simulink model "hnn_with_proof"  (R2024b)
settings: Solver=VariableStepAuto  StartTime=0.0  StopTime=10.0  RelTol=1e-3
settings Model: Creator=merlin  LastModifiedBy=merlin

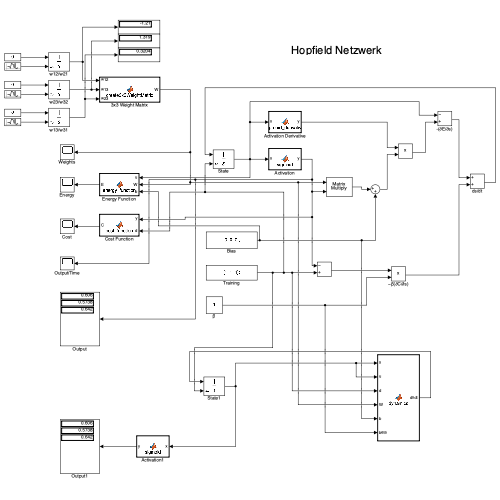
[thumbnail: Simulink's stored preview of the top-level diagram]
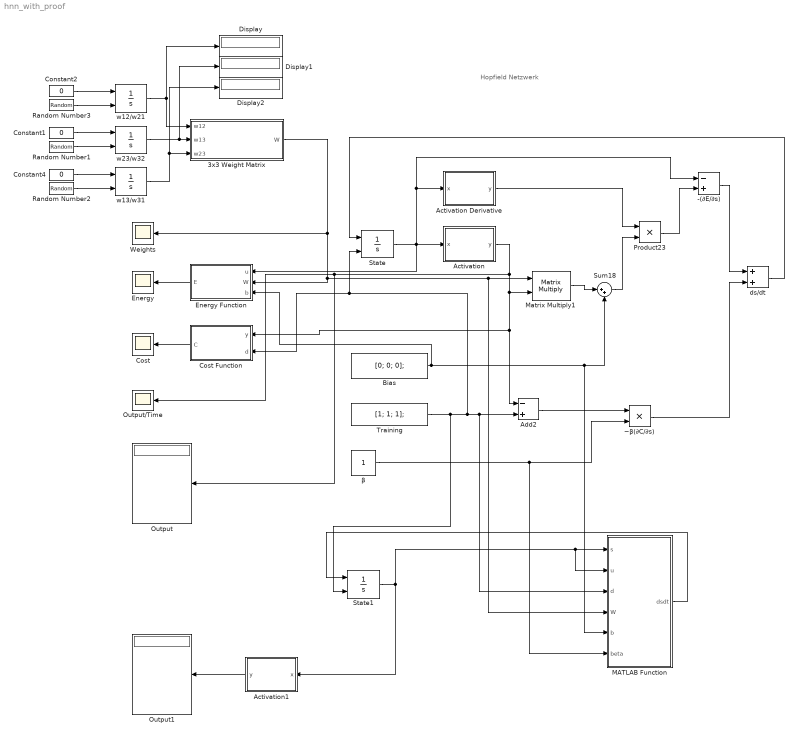
== system hnn_with_proof ==
  note: Hopfield Netzwerk
  -(∂E/∂s) : Sum  Inputs=-+
  3x3 Weight Matrix : MATLAB Function  TreatAsAtomicUnit=on
  Activation : MATLAB Function  TreatAsAtomicUnit=on
  Activation Derivative : MATLAB Function  TreatAsAtomicUnit=on
  Activation1 : MATLAB Function  TreatAsAtomicUnit=on
  Add2 : Sum  Inputs=-+
  Bias : Constant  Value=[0; 0; 0];  VectorParams1D=off
  Constant1 : Constant  Value=0
  Constant2 : Constant  Value=0
  Constant4 : Constant  Value=0
  Cost : Scope
  Cost Function : MATLAB Function  TreatAsAtomicUnit=on
  Display : Display
  Display1 : Display
  Display2 : Display
  Energy : Scope
  Energy Function : MATLAB Function  TreatAsAtomicUnit=on
  MATLAB Function : MATLAB Function  TreatAsAtomicUnit=on
  Matrix Multiply1 : Product  Multiplication=Matrix(*)
  Output : Display
  Output/Time : Scope
  Output1 : Display
  Product23 : Product
  Random Number1 : RandomNumber  Seed=23  SampleTime=0.1
  Random Number2 : RandomNumber  Seed=13  SampleTime=0.1
  Random Number3 : RandomNumber  Seed=12  SampleTime=0.1
  State : Integrator  InitialConditionSource=external
  State1 : Integrator  InitialConditionSource=external
  Sum18 : Sum  Inputs=|++
  Training : Constant  Value=[1; 1; 1];  VectorParams1D=off
  Weights : Scope
  ds/dt : Sum
  w12/w21 : Integrator  InitialConditionSource=external
  w13/w31 : Integrator  InitialConditionSource=external
  w23/w32 : Integrator  InitialConditionSource=external
  β : Constant  VectorParams1D=off
  −β(∂C/∂s) : Product
  wires:
  w12/w21/1 -> 3x3 Weight Matrix/1(w12), Display/1
  Constant4/1 -> w13/w31/1
  Random Number2/1 -> w13/w31/2
  Bias/1 -> MATLAB Function/5(b), Sum18/2, Energy Function/3(b)
  ds/dt/1 -> State/1
  Energy Function/1(E) -> Energy/1
  State/1 -> Activation/1(x), Energy Function/1(u), Activation Derivative/1(x), -(∂E/∂s)/1
  β/1 -> MATLAB Function/6(beta), −β(∂C/∂s)/2
  Training/1 -> State1/2, Cost Function/2(d), State/2, MATLAB Function/3(d), Add2/2
  Activation/1(y) -> Output/Time/1, Output/1, Cost Function/1(y), Add2/1, Matrix Multiply1/2
  -(∂E/∂s)/1 -> ds/dt/1
  Add2/1 -> −β(∂C/∂s)/1
  Matrix Multiply1/1 -> Sum18/1
  Activation Derivative/1(y) -> Product23/1
  Sum18/1 -> Product23/2
  −β(∂C/∂s)/1 -> ds/dt/2
  Cost Function/1(C) -> Cost/1
  Product23/1 -> -(∂E/∂s)/2
  3x3 Weight Matrix/1(W) -> Weights/1, Energy Function/2(W), MATLAB Function/4(W), Matrix Multiply1/1
  Constant2/1 -> w12/w21/1
  Random Number3/1 -> w12/w21/2
  Constant1/1 -> w23/w32/1
  Random Number1/1 -> w23/w32/2
  MATLAB Function/1(dsdt) -> State1/1
  State1/1 -> MATLAB Function/2(u), MATLAB Function/1(s), Activation1/1(x)
  Activation1/1(y) -> Output1/1
  w23/w32/1 -> Display1/1, 3x3 Weight Matrix/2(w13)
  w13/w31/1 -> Display2/1, 3x3 Weight Matrix/3(w23)

== matlab function hnn_with_proof/Cost Function ==
  data: y input; C output; d input
function C = cost_function(y, d)
    C = 0.5 * sum((y - d).^2);
end

== matlab function hnn_with_proof/3x3 Weight Matrix ==
  data: w12 input; W output; w13 input; w23 input
function W = create3x3WeightMatrix(w12, w13, w23)
    W = [0,    w12,  w13;
         w12,  0,    w23;
         w13,  w23,  0];
end

== matlab function hnn_with_proof/Energy Function ==
  data: u input; E output; W input; b input
function E = energy_function(u, W, b)
    rho = @(x) 1 ./ (1 + exp(-x));

    E = (1/2) * sum(u.^2) ...
        - (1/2) * sum(sum(W .* (rho(u) * rho(u)')))
        - sum(b .* rho(u));
end

== matlab function hnn_with_proof/MATLAB Function ==
  data: s input; u input; dsdt output; d input; W input; b input; beta input
function dsdt = dynamics(s, u, d, W, b, beta)
    rho       = @(x) 1./(1 + exp(-x));
    rho_prime = @(x) rho(x) .* (1 - rho(x));
    W_eff = W - diag(diag(W));
    energy_term = rho_prime(s) .* (W_eff * rho(u) + b);
    cost_term = beta * (d - rho(u));
    dsdt = energy_term - s + cost_term;
end

== matlab function hnn_with_proof/Activation1 ==
  data: x input; y output
function y = sigmoid(x)
y = 1 ./ (1 + exp(-x));
end

== matlab function hnn_with_proof/Activation Derivative ==
  data: x input; y output
function y = sigmoid_derivative(x)
sigmoid = 1 ./ (1 + exp(-x));
y = sigmoid .* (1 - sigmoid);
end

== matlab function hnn_with_proof/Activation ==
  data: x input; y output
function y = sigmoid(x)
y = 1 ./ (1 + exp(-x));
end
